simulink model "All_injectors_LQG_just_ss_model"  (R2022a)
settings: Solver=FixedStepAuto  StartTime=0.0  StopTime=RunTime  FixedStep=SampleTime  RelTol=1e-3
values from neighbouring files (symbols this model uses):
  K_vacuum = lqr(sysc_vacuum,Q_cost(1:12,1:12),R_cost)    [All_injectors_LQG_bop_ss_model_code.m]    (also in All_injectors_LQG_continuous_time_code.m; All_injectors_LQG_plasma_7_15_24_code.m; All_injectors_LQG_plasma_ss_model_code.m; Plasma_ss_model_new.m = load('lqr_gain_vacuum.mat').K_vacuum)
  SampleTime = 1e-7    (= 1e-07)    [All_injectors_LQG_bop_plasma_ss_model_code.m]    (also in All_injectors_LQG_bop_ss_model_code.m; All_injectors_LQG_continuous_time_code.m; All_injectors_LQG_plasma_7_15_24_code.m; All_injectors_LQG_plasma_ss_model_code.m)
  sys_d_vacuum = load("sys_d_vacuum.mat").sys_d    [All_injectors_LQG_bop_ss_model_code.m]    (also in All_injectors_LQG_continuous_time_code.m; All_injectors_LQG_plasma_7_15_24_code.m; All_injectors_LQG_plasma_ss_model_code.m; Plasma_ss_model_new.m)
  syskf_vacuum = load('syskf_vacuum.mat').syskf_vacuum    [Plasma_ss_model_new.m]
libraries: simulink x1
settings Model: Creator=ducks  LastModifiedBy=ducks
settings DataIOCC: ExternalInput=[t,V]

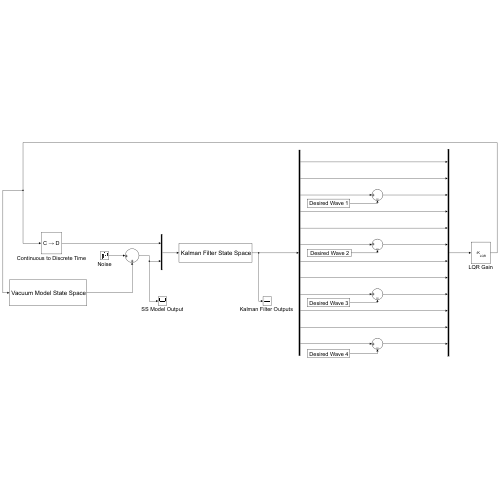
[thumbnail: Simulink's stored preview of the top-level diagram]
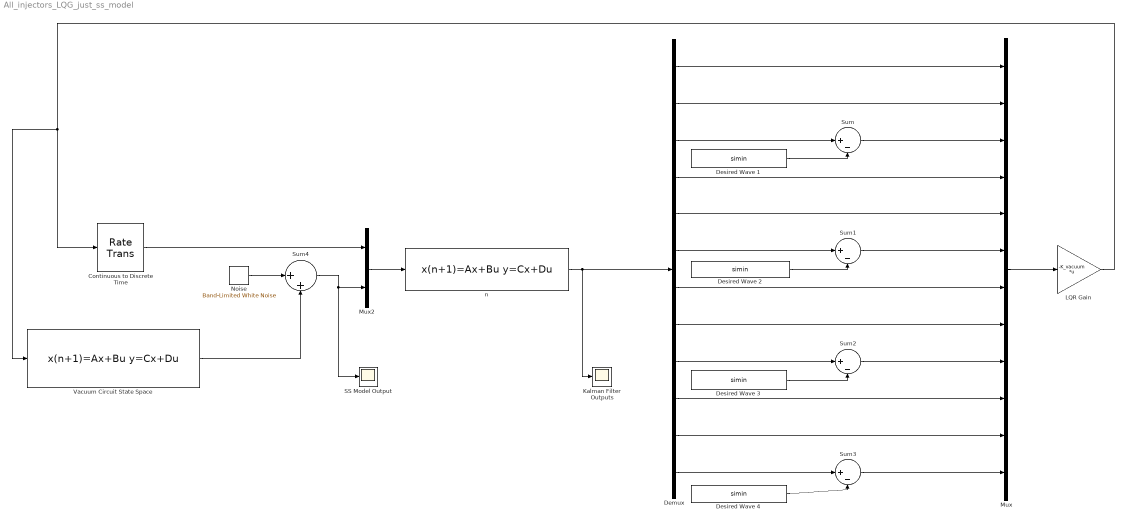
== system All_injectors_LQG_just_ss_model ==
  Continuous to Discrete Time : RateTransition  OutPortSampleTimeOpt=Inherit
      mask Display: disp('C \rightarrow D','texmode','on');
  Demux : Demux  Outputs=12
  Desired Wave {1..4} (4 alike) : FromWorkspace  VariableName=simin
      Desired Wave 1 mask Display: disp('\fontsize{20} Desired Wave 1','texmode','on');
      Desired Wave 2 mask Display: disp('\fontsize{20} Desired Wave 2','texmode','on');
      Desired Wave 3 mask Display: disp('\fontsize{20} Desired Wave 3','texmode','on');
      Desired Wave 4 mask Display: disp('\fontsize{20} Desired Wave 4','texmode','on')
  "Kalman Filter Outputs " : Scope
  LQR Gain : Gain  Gain=-K_vacuum  Multiplication=Matrix(K*u) (u vector)
      mask Display: disp('\fontsize{14} -K_{LQR}','texmode','on')
  Mux : Mux  Inputs=12
  Mux2 : Mux  Inputs=2
  Noise : simulink/Sources/Band-Limited White Noise  Cov=NoisePower  Ts=SampleTime  seed=[23341]
  SS Model Output : Scope
  Sum{,1..3} (4 alike) : Sum  Inputs=|+-
  Sum4 : Sum  Inputs=|++
  Vacuum Circuit State Space : DiscreteStateSpace  A=sys_d_vacuum.A  B=sys_d_vacuum.B  C=sys_d_vacuum.C  D=sys_d_vacuum.D  SampleTime=-1
      mask Display: disp('\fontsize{22} Vacuum Model State Space','texmode','on');
  n : DiscreteStateSpace  A=syskf_vacuum.A  B=syskf_vacuum.B  C=syskf_vacuum.C  D=syskf_vacuum.D  SampleTime=-1
      mask Display: disp('\fontsize{22} Kalman Filter State Space','texmode','on');
  wires:
  Desired Wave 3/1 -> Sum2/2
  n/1 -> Demux/1, "Kalman Filter Outputs "/1
  Desired Wave 2/1 -> Sum1/2
  Desired Wave 1/1 -> Sum/2
  Desired Wave 4/1 -> Sum3/2
  Vacuum Circuit State Space/1 -> Sum4/2
  Continuous to Discrete Time/1 -> Mux2/1
  Mux2/1 -> n/1
  Noise/1 -> Sum4/1
  Sum4/1 -> SS Model Output/1, Mux2/2
  LQR Gain/1 -> Continuous to Discrete Time/1, Vacuum Circuit State Space/1
  Demux/1 -> Mux/1
  Demux/2 -> Mux/2
  Demux/5 -> Mux/5
  Demux/7 -> Mux/7
  Demux/8 -> Mux/8
  Demux/10 -> Mux/10
  Demux/11 -> Mux/11
  Demux/3 -> Sum/1
  Sum/1 -> Mux/3
  Demux/4 -> Mux/4
  Demux/6 -> Sum1/1
  Sum1/1 -> Mux/6
  Demux/9 -> Sum2/1
  Sum2/1 -> Mux/9
  Demux/12 -> Sum3/1
  Sum3/1 -> Mux/12
  Mux/1 -> LQR Gain/1
